simulink model "cascade_realisation"  (R2020b)
settings: Solver=VariableStepAuto  StartTime=0.0  StopTime=10.0  RelTol=1e-3
settings Model: Creator=Arvind Hishikar  LastModifiedBy=Arvind Hishikar
settings DataIOCC: SaveOutput=off  SaveTime=off

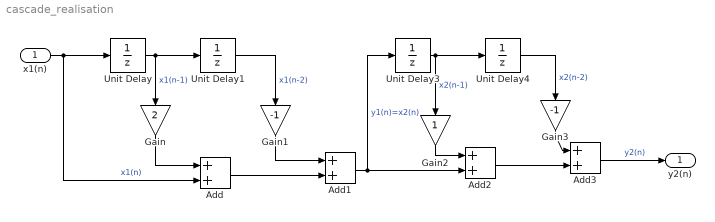
== system cascade_realisation ==
  x1(n) : Inport  OutDataTypeStr=double  PortDimensions=1  SampleTime=[0,1]
  Add{,1..3} (4 alike) : Sum
  Gain : Gain  Gain=2
  Gain1 : Gain  Gain=-1
  Gain2 : Gain
  Gain3 : Gain  Gain=-1
  Unit Delay{,1,3..4} (4 alike) : UnitDelay  SampleTime=-1  HasFrameUpgradeWarning=on
  y2(n) : Outport  OutDataTypeStr=double  PortDimensions=1  SampleTime=[0,1]
  wires:
  Unit Delay3/1 -> Gain2/1, Unit Delay4/1  "x2(n-1)"
  Unit Delay/1 -> Gain/1, Unit Delay1/1  "x1(n-1)"
  Gain2/1 -> Add2/1
  Add1/1 -> Unit Delay3/1, Add2/2  "y1(n)=x2(n)"
  x1(n)/1 -> Unit Delay/1, Add/2  "x1(n)"
  Unit Delay1/1 -> Gain1/1  "x1(n-2)"
  Gain3/1 -> Add3/1
  Gain1/1 -> Add1/1
  Add/1 -> Add1/2
  Gain/1 -> Add/1
  Add2/1 -> Add3/2
  Unit Delay4/1 -> Gain3/1  "x2(n-2)"
  Add3/1 -> y2(n)/1  "y2(n)"
